simulink model "tich_phan"  (R2016a)
settings: Solver=VariableStepAuto  StartTime=0.0  StopTime=10.0  RelTol=1e-3
settings Model: Creator=vuduc  LastModifiedBy=vuduc

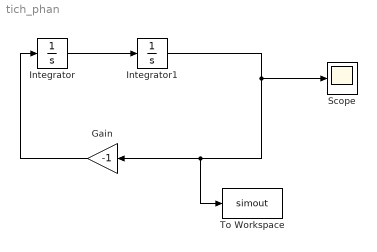
== system tich_phan ==
  Gain : Gain  Gain=-1
  Integrator : Integrator  InitialCondition=1
  Integrator1 : Integrator
  Scope : Scope
  To Workspace : ToWorkspace  VariableName=simout  SaveFormat=Timeseries  SampleTime=-1
  wires:
  Integrator1/1 -> To Workspace/1, Gain/1, Scope/1
  Integrator/1 -> Integrator1/1
  Gain/1 -> Integrator/1
